simulink model "model_with_b"  (R2019b)
settings: Solver=VariableStepAuto  StartTime=0.0  StopTime=0.5  RelTol=1e-3
values from neighbouring files (symbols this model uses):
  b = k*i_noload/w_noload    (= 6.57580978874e-08)    [DPT.m]
  J = 8.16*10^(-8)    (= 8.16e-08)    [DPT.m]
  k = 16.3*10^(-3)    (= 0.0163)    [DPT.m]
  L = 2.61*10^(-3)    (= 0.00261)    [DPT.m]
  R = 76.2    [DPT.m]
settings Model: Creator=катюшка  LastModifiedBy=катюшка

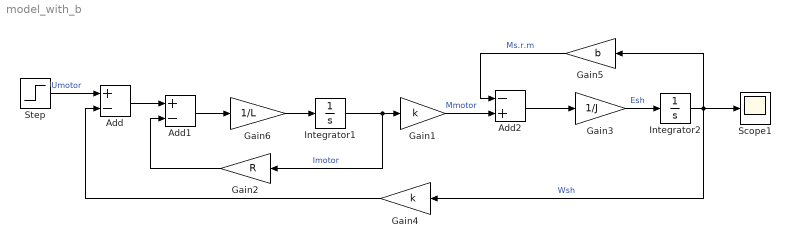
== system model_with_b ==
  Add : Sum  Inputs=+-
  Add1 : Sum  Inputs=+-
  Add2 : Sum  Inputs=-+
  Gain1 : Gain  Gain=k
  Gain2 : Gain  Gain=R
  Gain3 : Gain  Gain=1/J
  Gain4 : Gain  Gain=k
  Gain5 : Gain  Gain=b
  Gain6 : Gain  Gain=1/L
  Integrator1 : Integrator
  Integrator2 : Integrator
  Scope1 : Scope
  Step : Step  Time=0  After=24  SampleTime=0
  wires:
  Add/1 -> Add1/1
  Gain2/1 -> Add1/2
  Gain1/1 -> Add2/2  "Mmotor"
  Gain3/1 -> Integrator2/1  "Esh"
  Add2/1 -> Gain3/1
  Gain4/1 -> Add/2
  Integrator1/1 -> Gain2/1, Gain1/1  "Imotor"
  Add1/1 -> Gain6/1
  Step/1 -> Add/1  "Umotor"
  Gain5/1 -> Add2/1  "Ms.r.m"
  Gain6/1 -> Integrator1/1
  Integrator2/1 -> Scope1/1, Gain5/1, Gain4/1  "Wsh"
